simulink model "ALGO_Tanker_new_5Pin_baseline"  (R2023a)
settings: Solver=VariableStepAuto  StartTime=0  StopTime=60  RelTol=1e-3
StopFcn:
  | CompareSimResult_baseline
libraries: simulink x18, Solver_SF x1
(part 1 of 2)
CloseFcn:
  | rollover_simResult_save
settings Model: Creator=QXJ  LastModifiedBy=28303
settings SolverCC: AlgebraicLoopSolver=TrustRegion
settings DebuggingCC: UnconnectedInputMsg=warning  UnconnectedOutputMsg=warning  UnconnectedLineMsg=warning
settings ModelReferenceCC: EnableRefExpFcnMdlSchedulingChecks=on
settings SFSimCC: CustomCodeUndefinedFunction=UseInterfaceOnly

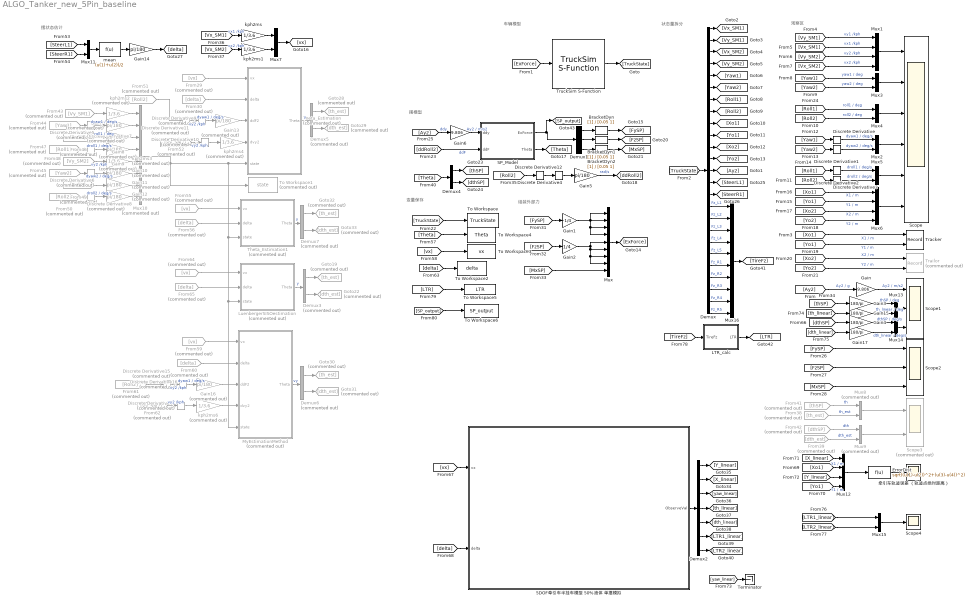
== system ALGO_Tanker_new_5Pin_baseline ==
  note: 摆状态估计
  note: 观察区
  note: 组装外部力
  note: 车辆模型
  note: 状态量拆分
  note: 变量保存
  note: 摆模型
  5DOF牵引车半挂车模型 50%液体 单摆模拟 : Subsystem
  BracketDyn : TransferFcn  Denominator=[0.05 1]
  BracketDyn1 : TransferFcn  Denominator=[0.05 1]
  BracketDyn2 : TransferFcn  Denominator=[0.05 1]
  Demux : Demux  Outputs=25
  Demux1 : Demux  Outputs=3
  Demux2 : Demux  Outputs=7
  Demux{3,5..7} (4 alike) : Demux  Commented=on  Outputs=2
  Demux4 : Demux  Outputs=2
  Discrete Derivative{,1..4,12} (6 alike) : simulink/Discrete/Discrete Derivative  gainval=1.0  ICPrevScaledInput=0.0  OutMin=[]  OutMax=[]  OutDataType=fixdt(1, 16)  OutScaling=2^-10  DoSatur=off
  Discrete Derivative{5..11,15..17} (10 alike) : simulink/Discrete/Discrete Derivative  Commented=on  gainval=1.0  ICPrevScaledInput=0.0  OutMin=[]  OutMax=[]  OutDataType=fixdt(1, 16)  OutScaling=2^-10  DoSatur=off
  ErrorDist : Fcn  Expr=sqrt((u(1)-u(2))^2+(u(3)-u(4))^2)
  From{29,55,59,64} (4 alike) : From  Commented=on  GotoTag=vx
  From{30,56,60,65} (4 alike) : From  Commented=on  GotoTag=delta
  From38 : From  Commented=on  GotoTag=th_est
  From39 : From  Commented=on  GotoTag=dth_est
  From41 : From  Commented=on  GotoTag=thSP
  From42 : From  Commented=on  GotoTag=dthSP
  From43 : From  Commented=on  GotoTag=Vy_SM1
  From44 : From  Commented=on  GotoTag=Yaw1
  From45 : From  Commented=on  GotoTag=Yaw2
  From46 : From  Commented=on  GotoTag=Roll1
  From47 : From  Commented=on  GotoTag=Roll1
  From48 : From  Commented=on  GotoTag=Vy_SM2
  From{49..51,61} (4 alike) : From  Commented=on  GotoTag=Roll2
  From52 : From  Commented=on  GotoTag=Vy_SM2
  From62 : From  Commented=on  GotoTag=Vy_SM2
  Gain : Gain  Gain=9.806
  Gain1 : Gain  Gain=-1/4
  Gain{7..13,16} (8 alike) : Gain  Commented=on  Gain=pi/180
  Gain14 : Gain  Gain=pi/180
  Gain{3..4,15,17} (4 alike) : Gain  Gain=180/pi
  Gain2 : Gain  Gain=1/4
  Gain5 : Gain  Gain=pi/180
  Gain6 : Gain  Gain=9.806
  Goto{19,28,30,32} (4 alike) : Goto  Commented=on  GotoTag=th_est
  Goto{22,29,31,33} (4 alike) : Goto  Commented=on  GotoTag=dth_est
  "LTR_calc " : MATLAB Function  TreatAsAtomicUnit=on
  LuenbergerSISOestimation : MATLAB Function  Commented=on  TreatAsAtomicUnit=on  SystemSampleTime=0.005
  Mux : Mux  Inputs=9
  Mux1 : Mux
  Mux10 : Mux  Commented=on  Inputs=8
  Mux{2..5,7,11,13..15} (9 alike) : Mux  Inputs=2
  Mux12 : Mux
  Mux16 : Mux  Inputs=10
  Mux6 : Mux
  Mux8 : Mux  Commented=on  Inputs=2
  Mux9 : Mux  Commented=on  Inputs=2
  MyEstimationMethod : MATLAB Function  Commented=on  TreatAsAtomicUnit=on  SystemSampleTime=0.005
  SP_Model : MATLAB Function  TreatAsAtomicUnit=on  SystemSampleTime=0.005
  Scope : Scope  NumInputPorts=6
  Scope1 : Scope  NumInputPorts=3
  Scope2 : Scope  NumInputPorts=3
  Scope3 : Scope  Commented=on  NumInputPorts=2
  Scope4 : Scope
  Terminator : Terminator
  Theta_Estimation : MATLAB Function  Commented=on  TreatAsAtomicUnit=on  SystemSampleTime=0.005
  Theta_Estimation1 : MATLAB Function  Commented=on  TreatAsAtomicUnit=on  SystemSampleTime=0.005
  To Workspace : ToWorkspace  VariableName=TruckState  SaveFormat=Timeseries  SampleTime=-1
  To Workspace1 : ToWorkspace  Commented=on  VariableName=state  SaveFormat=Timeseries  SampleTime=-1
  To Workspace2 : ToWorkspace  VariableName=delta  SaveFormat=Timeseries  SampleTime=-1
  To Workspace3 : ToWorkspace  VariableName=vx  SaveFormat=Timeseries  SampleTime=-1
  To Workspace4 : ToWorkspace  VariableName=Theta  SaveFormat=Timeseries  SampleTime=-1
  To Workspace5 : ToWorkspace  VariableName=LTR  SaveFormat=Timeseries  SampleTime=-1
  To Workspace6 : ToWorkspace  VariableName=SP_output  SaveFormat=Timeseries  SampleTime=-1
  Tracker : Record  FileSettingsInternal="{\"entries\":[{\"content\":{\"excelSettings\":{\"content\":{},\"type\":\"Streamout.ExcelSettings\"}},\"type\":\"Streamout.FileSettingStorage\",\"uuid\":\"aec428b3-b5ab-4f46-9125-b809af92a2bd\"}],\"packageUris\":[\"http://schema.mathworks.com/mf0/streamout_blocks/R2020a\"],\"version\":\"1.0\"}"  Layout=[1 1]  SignalsInternal="{\"entries\":[{\"content\":{\"signals\":[{\"content\":{\"blockPath\":[\"ALGO_Tanker_new_5Pin_baseline/Tracker\"],\"dimensions\":[1],\"domain\":\"ALGO_Tanker_new_5Pin_baseline/Tracker\",\"lineColor\":\"#a2142f\",\"plots\":[1],\"port\":1,\"sid\":[\"\"],\"signalID\":43,\"signalName\":\"X1 / m\"},\"type\":\"RecordBlkView.Signal\",\"uuid\":\"2f24ed56-e542-44bd-9784-fd43ced1a2ad\"},{\"content\":{\"blockPath\":[\"ALGO_Tanker_new_5Pin_baseline/Tracker\"],\"dimensions\":[1],\"domain\":\"ALGO_Tanker_new_5Pin_baseline/Tracker\",\"lineColor\":\"#139fff\",\"plots\":[1],\"port\":2,\"sid\":[\"\"],\"signalID\":47,\"signalName\":\"Y1 / m\"},\"type\":\"RecordBlkView.Signal\",\"uuid\":\"888b204b-f2f9-4a07-96ff-cc8a97ec0ab5\"}]},\"type\":\"RecordBlkView.InputSignals\",\"uuid\":\"7c72470c-5bbd-4b03-8b7f-21986a83b27f\"}],\"packageUris\":[\"http://schema.mathworks.com/mf0/streamout_blocks/R2020a\"],\"version\":\"1.0\"}"  VisualizationBindings="{\"xyplotplugin\":{\"info\":[{\"series\":[{\"bindingParametersList\":[{\"parameter\":\"X-Axis\",\"signalID\":43,\"signalName\":\"X1 \\/ m\"},{\"parameter\":\"Y-Axis\",\"signalID\":47,\"signalName\":\"Y1 \\/ m\"}],\"seriesID\":53818}],\"subplotID\":1}]}}"  CompatibilityTag=XY  st=-1
  "Trailor " : Record  Commented=on  FileSettingsInternal="{\"entries\":[{\"content\":{\"excelSettings\":{\"content\":{},\"type\":\"Streamout.ExcelSettings\"}},\"type\":\"Streamout.FileSettingStorage\",\"uuid\":\"42628413-2d8a-4dd7-9eb9-f9d26bce181c\"}],\"packageUris\":[\"http://schema.mathworks.com/mf0/streamout_blocks/R2020a\"],\"version\":\"1.0\"}"  Layout=[1 1]  SignalsInternal="{\"entries\":[{\"content\":{\"signals\":[{\"content\":{\"blockPath\":[\"ALGO_Tanker_new_5Pin_baseline/Trailor \"],\"dimensions\":[1],\"domain\":\"ALGO_Tanker_new_5Pin_baseline/Trailor \",\"lineColor\":\"#a2142f\",\"plots\":[1],\"port\":1,\"signalID\":16,\"signalName\":\"XY Graph:1\"},\"type\":\"RecordBlkView.Signal\",\"uuid\":\"6eea8f1e-a60b-4ba3-9267-a76fcc0df810\"},{\"content\":{\"blockPath\":[\"ALGO_Tanker_new_5Pin_baseline/Trailor \"],\"dimensions\":[1],\"domain\":\"ALGO_Tanker_new_5Pin_baseline/Trailor \",\"lineColor\":\"#139fff\",\"plots\":[1],\"port\":2,\"signalID\":19,\"signalName\":\"XY Graph:2\"},\"type\":\"RecordBlkView.Signal\",\"uuid\":\"9742e65f-64c3-4077-a878-ddc600cf04b1\"}]},\"type\":\"RecordBlkView.InputSignals\",\"uuid\":\"861e839e-7f05-49b0-87d7-e6303be47602\"}],\"packageUris\":[\"http://schema.mathworks.com/mf0/streamout_blocks/R2020a\"],\"version\":\"1.0\"}"  VisualizationBindings="{\"xyplotplugin\":{\"info\":[{\"series\":[{\"bindingParametersList\":[{\"parameter\":\"X-Axis\",\"signalID\":16,\"signalName\":\"XY Graph:1\"},{\"parameter\":\"Y-Axis\",\"signalID\":19,\"signalName\":\"XY Graph:2\"}],\"seriesID\":50861}],\"subplotID\":1}]}}"  CompatibilityTag=XY  st=-1
  TruckSim S-Function : Solver_SF/TruckSim S-Function  Priority=1  SIMFILE=ALGO_Tanker_TrajTrack_5Pin_Baseline.sim
      settings: SourceProductName=TruckSim S-Function
  kph2ms : Gain  Gain=1/3.6
  kph2ms1 : Gain  Gain=1/3.6
  kph2ms{2..4,6} (4 alike) : Gain  Commented=on  Gain=1/3.6
  mean : Fcn  Expr=(u(1)+u(2))/2
  牵引车轨迹误差 （轨迹点绝对距离） : Scope
  wires:
  kph2ms1/1 -> Mux7/2
  Mux7/1 -> [vx]
  kph2ms/1 -> Mux7/1
  From30/1 -> Theta_Estimation/2(delta)
  From29/1 -> Theta_Estimation/1(vx)
  [Vx_SM1] -> kph2ms/1  "vx1 /kph"
  [Vx_SM2] -> kph2ms1/1  "vx2 /kph"
  From45/1 -> Discrete Derivative6/1
  Discrete Derivative7/1 -> Gain9/1  "droll1 / deg/s"
  From47/1 -> Discrete Derivative7/1
  From50/1 -> Discrete Derivative8/1
  From43/1 -> kph2ms2/1
  From48/1 -> kph2ms3/1  "vy2 /kph"
  From44/1 -> Discrete Derivative5/1
  Discrete Derivative5/1 -> Gain7/1  "dyaw1 / deg/s"
  From46/1 -> Gain8/1  "roll1 / deg"
  Discrete Derivative6/1 -> Gain10/1  "dyaw2 / deg/s"
  From49/1 -> Gain11/1
  Discrete Derivative8/1 -> Gain12/1  "droll2 / deg/s"
  Gain12/1 -> Mux10/8
  Gain11/1 -> Mux10/7
  Gain10/1 -> Mux10/6
  kph2ms3/1 -> Mux10/5
  Gain9/1 -> Mux10/4
  Gain8/1 -> Mux10/3
  Gain7/1 -> Mux10/2
  kph2ms2/1 -> Mux10/1
  Discrete Derivative9/1 -> Gain13/1  "dyaw1 / deg/s"
  Discrete Derivative11/1 -> Discrete Derivative9/1  "vy2 /kph"
  From52/1 -> Discrete Derivative10/1  "vy2 /kph"
  Discrete Derivative10/1 -> kph2ms4/1
  From51/1 -> Discrete Derivative11/1
  Gain13/1 -> Theta_Estimation/3(ddF2)
  kph2ms4/1 -> Theta_Estimation/4(dvy2)
  [SteerL1] -> Mux11/1
  Mux11/1 -> mean/1
  [SteerR1] -> Mux11/2
  mean/1 -> Gain14/1
  Gain14/1 -> [delta]
  From55/1 -> Theta_Estimation1/1(vx)
  From56/1 -> Theta_Estimation1/2(delta)
  kph2ms6/1 -> MyEstimationMethod/4(dvy2)
  From62/1 -> Discrete Derivative17/1  "vy2 /kph"
  Discrete Derivative17/1 -> kph2ms6/1
  From61/1 -> Discrete Derivative15/1
  Gain16/1 -> MyEstimationMethod/3(ddF2)
  Discrete Derivative16/1 -> Gain16/1  "dyaw1 / deg/s"
  Discrete Derivative15/1 -> Discrete Derivative16/1  "vy2 /kph"
  From60/1 -> MyEstimationMethod/2(delta)
  From59/1 -> MyEstimationMethod/1(vx)
  Mux10/1 -> To Workspace1/1, Theta_Estimation/5(state), LuenbergerSISOestimation/3(state), MyEstimationMethod/5(state), Theta_Estimation1/3(state)
  MyEstimationMethod/1(Theta) -> Demux6/1  "vy"
  Demux3/1 -> Goto19/1
  Demux3/2 -> Goto22/1
  From64/1 -> LuenbergerSISOestimation/1(vx)
  From65/1 -> LuenbergerSISOestimation/2(delta)
  Theta_Estimation1/1(Theta) -> Demux7/1  "y"
  Demux5/2 -> Goto29/1
  Demux5/1 -> Goto28/1
  Theta_Estimation/1(Theta) -> Demux5/1  "y"
  LuenbergerSISOestimation/1(Theta) -> Demux3/1  "y"
  Demux6/2 -> Goto31/1
  Demux6/1 -> Goto30/1
  Demux7/2 -> Goto33/1
  Demux7/1 -> Goto32/1
  Discrete Derivative/1 -> Mux2/1  "dyaw1 / deg/s"
  Demux/12 -> [Yo2]
  Demux/11 -> [Xo2]
  [Xo1] -> Mux6/1  "X1 / m"
  TruckSim S-Function/1 -> [TruckState]
  [Xo2] -> "Trailor "/1  "X2 / m"
  Demux/1 -> [Vx_SM1]
  [TruckState] -> Demux/1
  [Yaw1] -> Mux3/1  "yaw1 / deg"
  [Yaw2] -> Mux3/2  "yaw2 / deg"
  Mux5/1 -> Scope/5
  Gain1/1 -> Mux/1, Mux/4, Mux/3, Mux/2
  [MxSP] -> Scope2/3
  [thSP] -> Gain3/1
  SP_Model/2(Theta) -> [Theta]
  Gain6/1 -> SP_Model/1(ddy)  "Ay2 / m/s2"
  [Vy_SM2] -> Mux1/3  "vy2 /kph"
  [Roll2] -> Mux4/2  "roll2 / deg"
  From39/1 -> Mux9/2  "dth_est"
  Demux4/1 -> [thSP]
  From38/1 -> Mux8/2  "th_est"
  Demux1/2 -> BracketDyn1/1
  Mux1/1 -> Scope/1
  [Theta] -> Demux4/1
  Demux/3 -> [Vx_SM2]
  Demux4/2 -> [dthSP]
  [Roll1] -> Mux4/1  "roll1 / deg"
  Mux4/1 -> Scope/3
  Gain4/1 -> Mux14/1  "dthSP / deg/s"
  BracketDyn/1 -> [FySP]
  BracketDyn1/1 -> [FzSP]
  Demux/2 -> [Vy_SM1]
  Gain5/1 -> [ddRoll2]  "rad/s"
  [Ay2] -> Gain6/1  "ddy"
  Discrete Derivative4/1 -> Discrete Derivative12/1
  [Roll2] -> Discrete Derivative4/1
  [Vx_SM2] -> Mux1/4  "vx2 /kph"
  [FySP] -> Gain1/1
  [Yaw1] -> Discrete Derivative/1
  SP_Model/1(ExForce) -> [SP_output], Demux1/1
  [Yo1] -> Mux6/2  "Y1 / m"
  [Roll1] -> Discrete Derivative2/1
  [Vx_SM1] -> Mux1/2  "vx1 /kph"
  Demux/9 -> [Xo1]
  [FzSP] -> Scope2/2
  [Yaw2] -> Discrete Derivative1/1
  [ExForce] -> TruckSim S-Function/1
  Demux1/1 -> BracketDyn/1
  Discrete Derivative2/1 -> Mux5/1  "droll1 / deg/s"
  From41/1 -> Mux8/1  "th"
  BracketDyn2/1 -> [MxSP]
  Demux/14 -> [SteerL1]
  Mux/1 -> [ExForce]
  [Roll2] -> Discrete Derivative3/1
  Mux6/1 -> Scope/6
  [Xo1] -> Tracker/1  "X1 / m"
  Demux/21 -> Mux16/6  "Fz_R1"
  Demux/22 -> Mux16/7  "Fz_R2"
  "LTR_calc "/1(LTR) -> [LTR]
  Mux9/1 -> Scope3/2
  Gain17/1 -> Mux14/2  "dth_linear / deg/s"
  Gain/1 -> Scope1/1  "Ay2 / m/s2"
  [TireFz] -> "LTR_calc "/1(TireFz)
  Demux/13 -> [Ay2]
  Demux/19 -> Mux16/4  "Fz_L4"
  Demux2/4 -> [th_linear]
  [dth_linear] -> Gain17/1
  Mux15/1 -> Scope4/1
  [Yo1] -> Tracker/2  "Y1 / m"
  Demux2/1 -> [Y_linear]
  Demux2/6 -> [LTR1_linear]
  5DOF牵引车半挂车模型 50%液体 单摆模拟/1(ObserveVal) -> Demux2/1
  [ddRoll2] -> SP_Model/2(ddF)  "ddF"
  Mux14/1 -> Scope1/3
  [yaw_linear] -> Terminator/1
  Mux2/1 -> Scope/4
  [Xo1] -> Mux12/2  "X1 / m"
  [Theta] -> To Workspace4/1
  [th_linear] -> Gain15/1
  Mux12/1 -> ErrorDist/1
  Demux/10 -> [Yo1]
  [Y_linear] -> Mux12/3
  Mux8/1 -> Scope3/1
  Demux2/7 -> [LTR2_linear]
  Demux/15 -> [SteerR1]
  Mux3/1 -> Scope/2
  Demux/6 -> [Yaw2]
  [Xo2] -> Mux6/3  "X2 / m"
  Demux2/2 -> [X_linear]
  [vx] -> To Workspace3/1
  [MxSP] -> Mux/9
  Demux/4 -> [Vy_SM2]
  Demux2/5 -> [dth_linear]
  [delta] -> 5DOF牵引车半挂车模型 50%液体 单摆模拟/2("delta ")
  Demux/7 -> [Roll1]
  [LTR2_linear] -> Mux15/2
  [dthSP] -> Gain4/1
  [vx] -> 5DOF牵引车半挂车模型 50%液体 单摆模拟/1(vx)
  [delta] -> To Workspace2/1
  Mux13/1 -> Scope1/2
  [Vy_SM1] -> Mux1/1  "vy1 /kph"
  [X_linear] -> Mux12/1
  ErrorDist/1 -> 牵引车轨迹误差 （轨迹点绝对距离）/1
  From42/1 -> Mux9/1  "dth"
  [Yo2] -> "Trailor "/2  "Y2 / m"
  [SP_output] -> To Workspace6/1
  Gain3/1 -> Mux13/1  "thSP / deg"
  Demux/8 -> [Roll2]
  Mux16/1 -> [TireFz]
  Gain15/1 -> Mux13/2  "th_linear / deg"
  [FzSP] -> Gain2/1
  Demux/5 -> [Yaw1]
  [Ay2] -> Gain/1  "Ay2 / g"
  Demux/17 -> Mux16/2  "Fz_L2"
  [Yo2] -> Mux6/4  "Y2 / m"
  Discrete Derivative1/1 -> Mux2/2  "dyaw2 / deg/s"
  [Yo1] -> Mux12/4  "Y1 / m"
  [LTR] -> To Workspace5/1
  [LTR1_linear] -> Mux15/1
  [FySP] -> Scope2/1
  Discrete Derivative3/1 -> Mux5/2  "droll2 / deg/s"
  Demux/16 -> Mux16/1  "Fz_L1"
  Demux1/3 -> BracketDyn2/1
  Discrete Derivative12/1 -> Gain5/1
  Gain2/1 -> Mux/8, Mux/7, Mux/6, Mux/5
  Demux/24 -> Mux16/9  "Fz_R4"
  Demux/20 -> Mux16/5  "Fz_L5"
  Demux/23 -> Mux16/8  "Fz_R3"
  Demux/18 -> Mux16/3  "Fz_L3"
  Demux2/3 -> [yaw_linear]
  Demux/25 -> Mux16/10  "Fz_R5"
  [TruckState] -> To Workspace/1

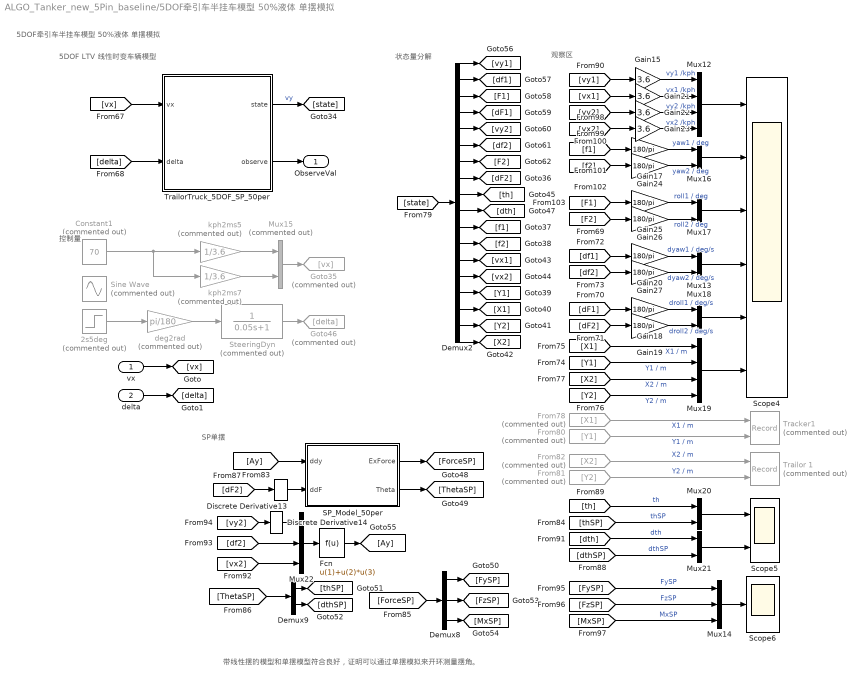
== system ALGO_Tanker_new_5Pin_baseline/5DOF牵引车半挂车模型 50%液体 单摆模拟 ==
  note: SP单摆
  note: 带线性摆的模型和单摆模型符合良好，证明可以通过单摆模拟来开环测量摆角。
  note: 控制量
  note: 5DOF牵引车半挂车模型 50%液体 单摆模拟
  note: 状态量分解
  note: 5DOF LTV 线性时变车辆模型
  note: 观察区
  vx : Inport
  "delta " : Inport  Port=2
  2s5deg : Step  Commented=on  Time=2  After=5  SampleTime=0
  Constant1 : Constant  Commented=on  Value=70
  Demux2 : Demux  Outputs=18
  Demux8 : Demux  Outputs=3
  Demux9 : Demux  Outputs=2
  Discrete Derivative13 : simulink/Discrete/Discrete Derivative  gainval=1.0  ICPrevScaledInput=0.0  OutMin=[]  OutMax=[]  OutDataType=fixdt(1, 16)  OutScaling=2^-10  DoSatur=off
  Discrete Derivative14 : simulink/Discrete/Discrete Derivative  gainval=1.0  ICPrevScaledInput=0.0  OutMin=[]  OutMax=[]  OutDataType=fixdt(1, 16)  OutScaling=2^-10  DoSatur=off
  Fcn : Fcn  Expr=u(1)+u(2)*u(3)
  From78 : From  Commented=on  GotoTag=X1
  From80 : From  Commented=on  GotoTag=Y1
  From81 : From  Commented=on  GotoTag=Y2
  From82 : From  Commented=on  GotoTag=X2
  Gain{15,21..23} (4 alike) : Gain  Gain=3.6
  Gain{17..20,24..27} (8 alike) : Gain  Gain=180/pi
  Goto35 : Goto  Commented=on  GotoTag=vx
  Goto46 : Goto  Commented=on  GotoTag=delta
  Mux12 : Mux
  Mux{13,16..18,20..21} (6 alike) : Mux  Inputs=2
  Mux14 : Mux  Inputs=3
  Mux15 : Mux  Commented=on  Inputs=2
  Mux19 : Mux
  Mux22 : Mux  Inputs=3
  SP_Model_50per : MATLAB Function  TreatAsAtomicUnit=on  SystemSampleTime=0.005
  Scope4 : Scope  NumInputPorts=6
  Scope5 : Scope  NumInputPorts=2
  Scope6 : Scope
  Sine Wave : Sin  Commented=on  Amplitude=25  Frequency=2*pi*0.2  SampleTime=0
  SteeringDyn : TransferFcn  Commented=on  Denominator=[0.05 1]
  Tracker1 : Record  Commented=on  FileSettingsInternal="{\"entries\":[{\"content\":{\"excelSettings\":{\"content\":{},\"type\":\"Streamout.ExcelSettings\"}},\"type\":\"Streamout.FileSettingStorage\",\"uuid\":\"a90f987a-d528-48a3-b948-a80540f660a2\"}],\"packageUris\":[\"http://schema.mathworks.com/mf0/streamout_blocks/R2020a\"],\"version\":\"1.0\"}"  Layout=[1 1]  SignalsInternal="{\"entries\":[{\"content\":{\"signals\":[{\"content\":{\"blockPath\":[\"ALGO_Tanker_new_5Pin_baseline/5DOF牵引车半挂车模型 50%液体 单摆模拟/Tracker1\"],\"dimensions\":[1],\"domain\":\"ALGO_Tanker_new_5Pin_baseline/5DOF￧ﾉﾵ￥ﾼﾕ￨ﾽﾦ￥ﾍﾊ￦ﾌﾂ￨ﾽﾦ￦ﾨﾡ￥ﾞﾋ 50%￦ﾶﾲ￤ﾽﾓ ￥ﾍﾕ￦ﾑﾆ￦ﾨﾡ￦ﾋﾟ/Tracker1\",\"lineColor\":\"#a2142f\",\"plots\":[1],\"port\":1,\"signalID\":24,\"signalName\":\"XY Graph:1\"},\"type\":\"RecordBlkView.Signal\",\"uuid\":\"3ed66f4e-d292-443a-9652-1644885d5cf5\"},{\"content\":{\"blockPath\":[\"ALGO_Tanker_new_5Pin_baseline/5DOF牵引车半挂车模型 50%液体 单摆模拟/Tracker1\"],\"dimensions\":[1],\"domain\":\"ALGO_Tanker_new_5Pin_baseline/5DOF￧ﾉﾵ￥ﾼﾕ￨ﾽﾦ￥ﾍﾊ￦ﾌﾂ￨ﾽﾦ￦ﾨﾡ￥ﾞﾋ 50%￦ﾶﾲ￤ﾽﾓ ￥ﾍﾕ￦ﾑﾆ￦ﾨﾡ￦ﾋﾟ/Tracker1\",\"lineColor\":\"#139fff\",\"plots\":[1],\"port\":2,\"signalID\":27,\"signalName\":\"XY Graph:2\"},\"type\":\"RecordBlkView.Signal\",\"uuid\":\"03e0ba51-6389-48fb-8d2a-e503b4cbd9e5\"}]},\"type\":\"RecordBlkView.InputSignals\",\"uuid\":\"2c6dba3d-ae40-4061-a45b-5c20937c901b\"}],\"packageUris\":[\"http://schema.mathworks.com/mf0/streamout_blocks/R2020a\"],\"version\":\"1.0\"}"  VisualizationBindings="{\"xyplotplugin\":{\"info\":[{\"series\":[{\"bindingParametersList\":[{\"parameter\":\"X-Axis\",\"signalID\":24,\"signalName\":\"XY Graph:1\"},{\"parameter\":\"Y-Axis\",\"signalID\":27,\"signalName\":\"XY Graph:2\"}],\"seriesID\":47850}],\"subplotID\":1}]}}"  CompatibilityTag=XY  st=-1
  Trailor 1 : Record  Commented=on  FileSettingsInternal="{\"entries\":[{\"content\":{\"excelSettings\":{\"content\":{},\"type\":\"Streamout.ExcelSettings\"}},\"type\":\"Streamout.FileSettingStorage\",\"uuid\":\"ee976611-5a1b-436c-9467-2f509ccfb164\"}],\"packageUris\":[\"http://schema.mathworks.com/mf0/streamout_blocks/R2020a\"],\"version\":\"1.0\"}"  Layout=[1 1]  SignalsInternal="{\"entries\":[{\"content\":{\"signals\":[{\"content\":{\"blockPath\":[\"ALGO_Tanker_new_5Pin_baseline/5DOF牵引车半挂车模型 50%液体 单摆模拟/Trailor 1\"],\"dimensions\":[1],\"domain\":\"ALGO_Tanker_new_5Pin_baseline/5DOF￧ﾉﾵ￥ﾼﾕ￨ﾽﾦ￥ﾍﾊ￦ﾌﾂ￨ﾽﾦ￦ﾨﾡ￥ﾞﾋ 50%￦ﾶﾲ￤ﾽﾓ ￥ﾍﾕ￦ﾑﾆ￦ﾨﾡ￦ﾋﾟ/Trailor 1\",\"lineColor\":\"#a2142f\",\"plots\":[1],\"port\":1,\"signalID\":32,\"signalName\":\"XY Graph:1\"},\"type\":\"RecordBlkView.Signal\",\"uuid\":\"54d57959-15ed-4e42-bd0f-8cbd995d0bf1\"},{\"content\":{\"blockPath\":[\"ALGO_Tanker_new_5Pin_baseline/5DOF牵引车半挂车模型 50%液体 单摆模拟/Trailor 1\"],\"dimensions\":[1],\"domain\":\"ALGO_Tanker_new_5Pin_baseline/5DOF￧ﾉﾵ￥ﾼﾕ￨ﾽﾦ￥ﾍﾊ￦ﾌﾂ￨ﾽﾦ￦ﾨﾡ￥ﾞﾋ 50%￦ﾶﾲ￤ﾽﾓ ￥ﾍﾕ￦ﾑﾆ￦ﾨﾡ￦ﾋﾟ/Trailor 1\",\"lineColor\":\"#139fff\",\"plots\":[1],\"port\":2,\"signalID\":35,\"signalName\":\"XY Graph:2\"},\"type\":\"RecordBlkView.Signal\",\"uuid\":\"095e148a-9d51-41f4-bd97-85008a41f26b\"}]},\"type\":\"RecordBlkView.InputSignals\",\"uuid\":\"4401373d-b9f0-4087-a766-ee8aa40abb39\"}],\"packageUris\":[\"http://schema.mathworks.com/mf0/streamout_blocks/R2020a\"],\"version\":\"1.0\"}"  VisualizationBindings="{\"xyplotplugin\":{\"info\":[{\"series\":[{\"bindingParametersList\":[{\"parameter\":\"X-Axis\",\"signalID\":32,\"signalName\":\"XY Graph:1\"},{\"parameter\":\"Y-Axis\",\"signalID\":35,\"signalName\":\"XY Graph:2\"}],\"seriesID\":49081}],\"subplotID\":1}]}}"  CompatibilityTag=XY  st=-1
  TrailorTruck_5DOF_SP_50per : MATLAB Function  TreatAsAtomicUnit=on  SystemSampleTime=0.01
  deg2rad : Gain  Commented=on  Gain=pi/180
  kph2ms5 : Gain  Commented=on  Gain=1/3.6
  kph2ms7 : Gain  Commented=on  Gain=1/3.6
  ObserveVal : Outport  VectorParamsAs1DForOutWhenUnconnected=off
  wires:
  Demux2/17 -> [Y2]
  [vx2] -> Mux22/3
  [vx1] -> Gain21/1
  [FzSP] -> Mux14/2  "FzSP"
  Mux16/1 -> Scope4/2
  Gain25/1 -> Mux17/1  "roll1 / deg"
  Mux17/1 -> Scope4/3
  [Y1] -> Mux19/2  "Y1 / m"
  [vy2] -> Gain22/1
  [state] -> Demux2/1
  From78/1 -> Tracker1/1  "X1 / m"
  Demux2/9 -> [th]
  [MxSP] -> Mux14/3  "MxSP"
  Demux2/18 -> [X2]
  Gain26/1 -> Mux17/2  "roll2 / deg"
  From81/1 -> Trailor 1/2  "Y2 / m"
  Mux14/1 -> Scope6/1
  Gain21/1 -> Mux12/2  "vx1 /kph"
  SteeringDyn/1 -> Goto46/1
  [dF2] -> Gain19/1
  [f2] -> Gain24/1
  [dF1] -> Gain18/1
  [vx2] -> Gain23/1
  [F2] -> Gain26/1
  Demux2/7 -> [F2]
  From80/1 -> Tracker1/2  "Y1 / m"
  Demux2/14 -> [vx2]
  Demux2/11 -> [f1]
  Gain27/1 -> Mux13/2  "dyaw2 / deg/s"
  [df1] -> Gain20/1
  2s5deg/1 -> deg2rad/1
  [F1] -> Gain25/1
  [X1] -> Mux19/1  "X1 / m"
  Gain19/1 -> Mux18/2  "droll2 / deg/s"
  Gain18/1 -> Mux18/1  "droll1 / deg/s"
  Mux19/1 -> Scope4/6
  Demux8/3 -> [MxSP]
  [df2] -> Mux22/2
  Discrete Derivative14/1 -> Mux22/1
  Mux20/1 -> Scope5/1
  Gain15/1 -> Mux12/1  "vy1 /kph"
  Mux13/1 -> Scope4/4
  Gain23/1 -> Mux12/4  "vx2 /kph"
  [FySP] -> Mux14/1  "FySP"
  [vy1] -> Gain15/1
  Demux2/4 -> [dF1]
  Fcn/1 -> [Ay]
  Mux22/1 -> Fcn/1
  kph2ms5/1 -> Mux15/1
  [ThetaSP] -> Demux9/1
  Mux15/1 -> Goto35/1
  [dthSP] -> Mux21/2  "dthSP"
  [thSP] -> Mux20/2  "thSP"
  deg2rad/1 -> SteeringDyn/1
  Gain24/1 -> Mux16/2  "yaw2 / deg"
  Demux2/12 -> [f2]
  [X2] -> Mux19/3  "X2 / m"
  Discrete Derivative13/1 -> SP_Model_50per/2(ddF)
  Demux8/1 -> [FySP]
  Demux8/2 -> [FzSP]
  Gain17/1 -> Mux16/1  "yaw1 / deg"
  Gain20/1 -> Mux13/1  "dyaw1 / deg/s"
  [vy2] -> Discrete Derivative14/1
  Mux18/1 -> Scope4/5
  [ForceSP] -> Demux8/1
  SP_Model_50per/1(ExForce) -> [ForceSP]
  TrailorTruck_5DOF_SP_50per/1(state) -> [state]  "vy"
  [delta] -> TrailorTruck_5DOF_SP_50per/2(delta)
  [dF2] -> Discrete Derivative13/1
  [f1] -> Gain17/1
  Demux2/15 -> [Y1]
  Mux12/1 -> Scope4/1
  [vx] -> TrailorTruck_5DOF_SP_50per/1(vx)
  From82/1 -> Trailor 1/1  "X2 / m"
  Demux2/6 -> [df2]
  Demux2/2 -> [df1]
  kph2ms7/1 -> Mux15/2
  Demux2/5 -> [vy2]
  Demux2/3 -> [F1]
  [Ay] -> SP_Model_50per/1(ddy)
  SP_Model_50per/2(Theta) -> [ThetaSP]
  Demux2/8 -> [dF2]
  Demux9/1 -> [thSP]
  [Y2] -> Mux19/4  "Y2 / m"
  Demux2/16 -> [X1]
  Constant1/1 -> kph2ms7/1, kph2ms5/1
  Demux2/13 -> [vx1]
  Demux2/1 -> [vy1]
  Demux9/2 -> [dthSP]
  [df2] -> Gain27/1
  Mux21/1 -> Scope5/2
  [dth] -> Mux21/1  "dth"
  [th] -> Mux20/1  "th"
  Demux2/10 -> [dth]
  Gain22/1 -> Mux12/3  "vy2 /kph"
  vx/1 -> [vx]
  "delta "/1 -> [delta]
  TrailorTruck_5DOF_SP_50per/2(observe) -> ObserveVal/1

== matlab function ALGO_Tanker_new_5Pin_baseline/SP_Model ==
  data: ddy input; ExForce output; ddF input; Theta output
function [ExForce,Theta] = SP_Model(ddy,ddF)
persistent sim_param Ts y0
%% 定义摆
if isempty(Ts)
%SP模型，共5个参数拟合
% 参数 m1 h0 hp lp coeff
x=[10890,1.5,0.13,0.97,0.13];
% 获取参数
sim_param=getParam_SP(x);
%初始状态量
y0=zeros(9,1);
%采样时间
Ts=0.005;
end

y=y0;

%% 求解微分方程
dy=zeros(9,1);
dy(1)=y(2);
dy(2)=ddy;
dy(3)=(dy(2)-y(3))/Ts;
dy(4)=y(5);
dy(5)=ddF;
dy(6)=(dy(5)-y(6))/Ts;
dy(7)=y(8);
dy(8)=calc_ddth_SP(y,sim_param);
dy(9)=(dy(8)-y(9))/Ts;
y=y0+dy*Ts;
%% 计算三向力输出
[Fy,Fz,Mx]=calc_Fp_SP(y,sim_param);
ExForce=[Fy,Fz,Mx];
%% 更新状态量
y0=y;
th=y(7);
dth=y(8);
Theta=[th,dth];
end

%% 根据变量获取参数
function sim_param=getParam_SP(x)
%根据变量生成传输参数
TotMass=14462;
m1=x(1);%参数1
m0=TotMass-m1;
h0=x(2);%参数2
hp=x(3);%参数3
lp=x(4);%参数4
g=9.806;
coeff=x(5);%参数5
sim_param=[m0,m1,h0,hp,lp,g,coeff];
end

%% 求解三向力输出
function [Fy,Fz,Mx] = calc_Fp_SP(state,param)
% sim_param=[m0,m1,h0,hp,lp,g,coeff];
m0=param(1);
m1=param(2);
h0=param(3);
hp=param(4);
lp=param(5);
g=param(6);
% co=param(7);

% y=state(1);
% dy=state(2);
ddy=state(3);
f=state(4);
df=state(5);
ddf=state(6);
th=state(7);
dth=state(8);
ddth=state(9);

%定义运算符简写
sf=sin(f);
cf=cos(f);
s2=sin(th+f);
c2=cos(th+f);
L=lp+hp;
%定义质量块的 位置矢量
exh=0.77; %额外增加的高度是罐底到车轴心的高度
R0=[-(exh+h0)*sf,(exh+h0)*cf];

R1=[-(exh+L)*sf+lp*s2
    (exh+L)*cf-lp*c2];

ddRp0=[ddy-h0*cf*ddf+df^2*h0*sf
-h0*sf*ddf-h0*cf*df^2+g];

ddRp1=[ddy+ddf*(-L*cf+lp*c2)+ddth*(lp*c2)+df^2*(L*sf-lp*s2)+dth^2*(-lp*s2)+df*dth*(-2*lp*s2)
ddf*(-L*sf+lp*s2)+ddth*(lp*s2)+df^2*(-L*cf+lp*c2)+dth^2*(lp*c2)+df*dth*(2*lp*c2)+g];

Fp=m0*ddRp0+m1*ddRp1;
Fy=Fp(1)*cf-(-Fp(2))*sf;
Fz=(-Fp(2))*cf+Fp(1)*sf;
Mx0=(m0*(R0(1)*-ddRp0(2)+R0(2)*ddRp0(1)));
Mx1=(m1*(R1(1)*-ddRp1(2)+R1(2)*ddRp1(1)));

Mx=Mx0+Mx1;

end
%% 求解ddth
function ddth = calc_ddth_SP(state,param)
% sim_param=[m0,m1,h0,hp,lp,g,coeff];
% m0=param(1);
% m1=param(2);
% h0=param(3);
hp=param(4);
lp=param(5);
g=param(6);
co=param(7);

% y=state(1);
% dy=state(2);
ddy=state(3);
f=state(4);
df=state(5);
ddf=state(6);
th=state(7);
dth=state(8);
% ddth=state(9);


%定义运算符简写
s1=sin(th);
c1=cos(th);
s2=sin(th+f);
c2=cos(th+f);
L=lp+hp;

ddth=-(ddy*lp*c2+ddf*(-lp*L*c1+lp^2)-df^2*lp*L*s1+g*lp*s2)/(lp^2);
ddth=ddth-co*dth;

end

== matlab function ALGO_Tanker_new_5Pin_baseline/Theta_Estimation ==
  data: vx input; delta input; ddF2 input; dvy2 input; state input; Theta output
function Theta=Theta_Estimation(vx,delta,ddF2,dvy2,state)
%% 初始状态定义
%要记得设置本模块的采样时间哦
persistent Ts                             %采样时间
persistent th0 dth0 state0 lambda   %摆状态
if isempty(th0)
    Ts=0.005;
   th0=0;dth0=0; 
   state0=zeros(8,1);
   lambda=0.995;
end
%% 定义动力学模型参数
persistent a b c d e                    %轴距纵向几何参数
persistent h1 h2 hc1 hc2                %质心至侧倾轴线距离
                                        %铰接点至侧倾轴线距离
persistent m1 m2 m1s m2s g;g=9.806;
persistent I1zz I1xx I1xz I2zz I2xx I2xz %惯性参量
persistent k1 k2 k3                      %线性轮胎模型参数
persistent kr1 kr2 c1 c2 k12             %悬架模型参数
persistent m0 mp h0 hp lp co             %摆模型参数
if isempty(a)
%SP模型，共5个参数拟合
% 参数 m1 h0 hp lp coeff
x=[10890,1.5,0.13,0.97,0.13];
sim_param=getParam_SP(x);
% sim_param=[m0,m1,h0+0.77,hp+0.77,lp,g,coeff];
m0=sim_param(1);
mp=sim_param(2);
h0=sim_param(3);
hp=sim_param(4);
lp=sim_param(5);
co=sim_param(7);
%车辆模型参数
L1=(5+6.27)/2;L2=(10.15+11.5)/2;       %轴距平均
a=1.385;b=L1-a;c=5.635-a;e=5.5;d=L2-e; %纵向几何
hm1s=1.02; %牵引车质心高度
hm2s=1.58; %50%充液率时半挂车质心高度
hhitch=1.1;%交接点高度
hroll1=0.2314;hroll2=0.9630;                     %侧倾中心高度
h1=hm1s-hroll1;h2=hm2s-hroll2;hc1=hhitch-hroll1;hc2=hhitch-hroll2;%高度几何
m1s=6310;m1=m1s+570+785*2;             %牵引车质量
% m2s=5925;m2=m2s+665*2;                 %半挂车空载质量
m2s=20387;m2=m2s+665*2;
I1xx=6879;I1xz=130;I1zz=19665;         %牵引车惯量
% I2xx=9960;I2xz=0;I2zz=179992;          %半挂车惯量
I2xx=34652;I2xz=0;I2zz=331380;
%轮胎模型参数
k1=-37e4;k2=-82e4;k3=-80e4;             %侧偏刚度
kr1=18.7e5;kr2=9.14e5;k12=68.3e5;             %侧倾刚度
c1=64.4e3;c2=197.7e3;                        %悬架等效阻尼
end
%% 定义线性动力学模型
df2=state0(6);
dF2=state0(8);
vx1=vx(1);vx2=vx(2);
%线性车辆动力学模型
% M*dX = A0*X + B0*u
m14=-m1s*h1*c-I1xz;
m21=m1*vx1*hc1-m1s*h1*vx1;
m24=I1xx+2*m1s*h1^2-m1s*h1*hc1;
m55=m2*vx2*hc2-m2s*h2*vx2;
m58=I2xx+2*m2s*h2^2-m2s*h2*hc2;

M=[m1*vx1*c, I1zz, 0,   m14,     0,        0,   0,     0;
    m21,    -I1xz, 0,   m24,     0,        0,   0,     0;
   m1*vx1,      0, 0, -m1s*h1, m2*vx2,     0,   0, -m2s*h2;
     0,         0, 0,     0,  m2*vx2*e, -I2zz,  0, I2xz-m2s*h2*e;
     0,         0, 0,     0,    m55,    -I2xz,  0,    m58;
     1,    -c/vx1, 0, -hc1/vx1,  -1,   -e/vx2,  0, hc2/vx2;
     0,         0, 1,     0,     0,        0,   0,     0;
     0,         0, 0,     0,     0,        0,   1,     0   ];
 
 a11 = (c+a)*k1 + (c-b)*k2;
 a12 = a*(c+a)*k1/vx1 - b*(c-b)*k2/vx1 - m1*vx1*c;
 a22 = (a*k1-b*k2)*hc1/vx1 + (m1s*h1-m1*hc1)*vx1;
 a23 = m1s*g*h1 - kr1 -k12;
 a32 = (a*k1-b*k2)/vx1 - m1*vx1;
 a36 = -d*k3/vx2 - m2*vx2;
 a46 = -d*(e+d)*k3/vx2 - m2*vx2*e;
 a56 = (m2s*h2-m2*hc2)*vx2 - d*k3*hc2/vx2;
 a57 = m2s*g*h2 - kr2 -k12;
 %  X=   b1     df1    F1  dF1        b2  df2, F2   dF2 
 Acm0=[ a11,    a12,    0,   0,       0,   0,  0,    0;
   (k1+k2)*hc1, a22,  a23, -c1,       0,   0, k12,   0;
     k1+k2,     a32,    0,   0,      k3,  a36, 0,    0;
        0,       0,     0,   0, (e+d)*k3, a46, 0,    0;
        0,       0,    k12,  0, e*k3*h2, a56, a57, -c2;
        0,      -1,     0,   0,       0,   1,  0,    0;
        0,       0,     0,   1,       0,   0,  0,    0;
        0,       0,     0,   0,       0,   0,  0,    1   ];
    
 Bcm0=[-(c+a)*k1, -k1*hc1, -k1, 0, 0, 0, 0, 0]';

 %       1    2   3    4    5    6    7    8   9   10  11   12   13  14  15 16  17 18
%  X = vy1,  df1,F1, dF1, vy2, df2,  F2, dF2, f1, f2, vx1, vx2, Y1, X1, Y2,X2  th dth
% dX = dvy1;ddf1;dF1;ddF1;dvy2;ddf2;dF2;ddF2;df1;df2;dvx1;dvx2;dY1;dX1;dY2;dX2;dth;ddth
th=th0;dth=dth0;

M_=zeros(10);
M_(10,5)=cos(th)/lp;
M_(10,9)=co;
M_(10,10)=1;
M_(9,9)=1;
M_(3,:)=[0,0,0,0,m0-mp*(cos(th)^2-1),0,0,-h0*m0-mp*(hp+lp-lp),...
    -mp*(co*lp+2*dth*lp*sin(th)),0];
M_(4,:)=M_(3,:)*e;
M_(5,:)=M_(3,:)*hc2+...
[0,0,0,0,-h0*m0-hp*mp*sin(th)^2-lp*mp*sin(th)^2,0,-2*dF2*lp*mp*sin(th)*(hp+lp-lp),...
  m0*h0^2+mp*((hp+lp-lp)^2+lp^2*sin(th)^2),0,0];

%       1    2   3    4    5    6    7    8   17 18
%  X =  0,   0,  0,   0, vy2,   0,  F2, dF2,  th  0
% dX =  0,   0,  0,   0,  0;  ddf2; 0; ddF2;;dth;ddth 
A_=zeros(10);
A_(9,10)=1;
A_(10,6)=-(vx2)/lp;
a_317=mp*(ddF2*lp*sin(th)+(cos(th)*(g*lp-lp*sin(th)*(dvy2+df2*vx2)))...
    /lp+dth^2*lp-lp*sin(th)*(co*dth+(g*lp*sin(th)+lp*(dvy2+df2*vx2))/lp^2));
A_(3,:)=[ 0, 0, 0, 0, 0,-m0*vx2+mp*(vx2-vx2^2), 0, 0,a_317,0];
A_(4,:)=A_(3,:)*e;
A_(5,:)=A_(3,:)*hc2+...
[ 0, 0, 0, 0, 0, vx2*(h0*m0),0,2*dF2*lp*mp*sin(th)*(hp+lp-lp), ...
 mp*(dvy2*hp*sin(2*th)-g*hp*cos(2*th)-g*lp*cos(2*th)-dF2^2*lp^2*cos(2*th)-2*ddF2*lp^2*sin(th) ...
+dvy2*lp*sin(2*th)+dF2^2*lp^2-dth^2*lp^2-2*ddF2*hp*lp*sin(th)+dF2^2*hp*lp...
 -dth^2*hp*lp+co*dth*lp^2*sin(th)+df2*hp*vx2*sin(2*th)+df2*lp*vx2*sin(2*th)+co*dth*hp*lp*sin(th)),...
 -mp*(lp*(co+2*dth*sin(th))*(hp+lp-lp)+lp^2*sin(th)*(2*dth-co*sin(th)))];

%       1    2   3    4    5    6    7    8   9  10
%  X =  0,   0,  0,   0,   0, df2,   0,   0, th  0
% dX =  0;   0;  0;   0;dvy2;   0;dF2;ddF2;dth;  0
 Trans0=diag([vx1,1,1,1,vx2,1,1,1,1,1]);
 M_=Trans0*M_;
 A_=Trans0*A_;
 Acm=([M,zeros(8,2);zeros(2,10)]+M_)\([Acm0,zeros(8,2);zeros(2,10)]+A_);
 Bcm=([M,zeros(8,2);zeros(2,10)]+M_)\[Bcm0;zeros(2,1)];
 
 %% 增广状态量 并转变bi为vyi
 
 Trans=diag([1/vx1,1,1,1,1/vx2,1,1,1,1,1]);
 Ac=Trans*Acm;
 Bc=Trans*Bcm;
 
 %% 离散化线性模型
 [A,B]=c2d_zoh(Ac,Bc,Ts);             %离散化线性模型
 A0=A(1:8,1:8);
 A1=A(1:8,9:10);
 B0=B(1:8,1);
%       1   2    3    4   5    6    7    8   9  10
% dX=[dvy1;ddf1;dF1;ddF1;dvy2;ddf2;dF2;ddF2;th;dth];
%维度：10×1 
%% 进行状态估计
W=diag([20 10 20 1 20 20 20 1]);
Rho=diag([1.5 0.5])*0.0001;
Theta=(A1'*W*A1+Rho)\A1'*(state-A0*state0-B0*delta);

%% 保存状态量
th = RLS1(1,Theta(1),10,lambda);
dth0=(th-th0)/Ts;
th0=th;
% dth0 = RLS2(1,Theta(2),20,lambda);
% th0=Theta(1)*lambda+dth0*(1-lambda);dth0=Theta(2)*lambda+dth0*(1-lambda);
Theta(1)=th0;
Theta(2)=dth0;
state0=state;


end
function Fai = RLS1(fai_m1,Ym1,Nm,lambda)
persistent Pm_ Fai_ Ym fai_m
%初始赋值
if isempty(Pm_)
    Fai_=1e-10;
    Pm_=10*eye(Nm);
    Ym=ones(1,Nm)*1e-10;
    fai_m=ones(Nm,1);
end
%对fai_m 1xNm和 Ym 进行更新
fai_m(2:end)=fai_m(1:end-1);
Ym(2:end)=Ym(1:end-1);
fai_m(1)=fai_m1;
Ym(1)=Ym1;
%计算卡尔曼增益
K=Pm_*fai_m/(lambda+fai_m'*Pm_*fai_m);
%进行滤波
Fai=Fai_+(Ym-fai_m'*Fai_)*K;
%更新矩阵
Pm=1/lambda*(Pm_-K*fai_m'*Pm_);
Pm_=Pm;
Fai_=Fai;
end
function Fai = RLS2(fai_m1,Ym1,Nm,lambda)
persistent Pm_ Fai_ Ym fai_m
%初始赋值
if isempty(Pm_)
    Fai_=1e-10;
    Pm_=10*eye(Nm);
    Ym=ones(1,Nm)*1e-10;
    fai_m=ones(Nm,1);
end
%对fai_m 1xNm和 Ym 进行更新
fai_m(2:end)=fai_m(1:end-1);
Ym(2:end)=Ym(1:end-1);
fai_m(1)=fai_m1;
Ym(1)=Ym1;
%计算卡尔曼增益
K=Pm_*fai_m/(lambda+fai_m'*Pm_*fai_m);
%进行滤波
Fai=Fai_+(Ym-fai_m'*Fai_)*K;
%更新矩阵
Pm=1/lambda*(Pm_-K*fai_m'*Pm_);
Pm_=Pm;
Fai_=Fai;
end

%% 根据变量获取参数
function sim_param=getParam_SP(x)
%根据变量生成传输参数
TotMass=14462;
m1=x(1);%参数1
m0=TotMass-m1;
h0=x(2);%参数2
hp=x(3);%参数3
lp=x(4);%参数4
g=9.806;
coeff=x(5);%参数5
sim_param=[m0,m1,h0+0.77,hp+0.77,lp,g,coeff];
end

== matlab function ALGO_Tanker_new_5Pin_baseline/Theta_Estimation1 ==
  data: vx input; delta input; state input; Theta output
function Theta=Theta_Estimation(vx,delta,state)
%% 初始状态定义
%要记得设置本模块的采样时间哦
persistent Ts                            %采样时间
persistent th0 dth0 state0 lambda   %摆状态
if isempty(Ts)
   Ts=0.005;%采样时间
   %初始化状态量
   state0=zeros(2,1);
   lambda=0.995;
end
%% 定义动力学模型参数
persistent a b c d e                    %轴距纵向几何参数
persistent h1 h2 hc1 hc2                %质心至侧倾轴线距离
                                        %铰接点至侧倾轴线距离
persistent m1 m2 m1s m2s g;g=9.806;
persistent I1zz I1xx I1xz I2zz I2xx I2xz %惯性参量
persistent k1 k2 k3                      %线性轮胎模型参数
persistent kr1 kr2 c1 c2 k12             %悬架模型参数
persistent m0 mp h0 hp lp co             %摆模型参数
if isempty(a)
%SP模型，共5个参数拟合
% 参数 m1 h0 hp lp coeff
x=[10890,1.5,0.13,0.97,0.13];
sim_param=getParam_SP(x);
% sim_param=[m0,m1,h0+0.77,hp+0.77,lp,g,coeff];
m0=sim_param(1);
mp=sim_param(2);
h0=sim_param(3);
hp=sim_param(4);
lp=sim_param(5);
co=sim_param(7);
%车辆模型参数
L1=(5+6.27)/2;L2=(10.15+11.5)/2;       %轴距平均
a=1.385;b=L1-a;c=5.635-a;e=5.5;d=L2-e; %纵向几何
hm1s=1.02; %牵引车质心高度
hm2s=1.58; %50%充液率时半挂车质心高度
hhitch=1.1;%交接点高度
hroll1=0.2314;hroll2=0.9630;                     %侧倾中心高度
h1=hm1s-hroll1;h2=hm2s-hroll2;hc1=hhitch-hroll1;hc2=hhitch-hroll2;%高度几何
m1s=6310;m1=m1s+570+785*2;             %牵引车质量
% m2s=5925;m2=m2s+665*2;                 %半挂车空载质量
m2s=20387;m2=m2s+665*2;
I1xx=6879;I1xz=130;I1zz=19665;         %牵引车惯量
% I2xx=9960;I2xz=0;I2zz=179992;          %半挂车惯量
I2xx=34652;I2xz=0;I2zz=331380;
%轮胎模型参数
k1=-37e4;k2=-82e4;k3=-80e4;             %侧偏刚度
kr1=18.7e5;kr2=9.14e5;k12=68.3e5;             %侧倾刚度
c1=64.4e3;c2=197.7e3;                        %悬架等效阻尼
end
%% 定义线性动力学模型
vx1=vx(1);vx2=vx(2);dF2=state(8);
%线性车辆动力学模型
% M*dX = A0*X + B0*u
m14=-m1s*h1*c-I1xz;
m21=m1*vx1*hc1-m1s*h1*vx1;
m24=I1xx+2*m1s*h1^2-m1s*h1*hc1;
m55=m2*vx2*hc2-m2s*h2*vx2;
m58=I2xx+2*m2s*h2^2-m2s*h2*hc2;

M=[m1*vx1*c, I1zz, 0,   m14,     0,        0,   0,     0;
    m21,    -I1xz, 0,   m24,     0,        0,   0,     0;
   m1*vx1,      0, 0, -m1s*h1, m2*vx2,     0,   0, -m2s*h2;
     0,         0, 0,     0,  m2*vx2*e, -I2zz,  0, I2xz-m2s*h2*e;
     0,         0, 0,     0,    m55,    -I2xz,  0,    m58;
     1,    -c/vx1, 0, -hc1/vx1,  -1,   -e/vx2,  0, hc2/vx2;
     0,         0, 1,     0,     0,        0,   0,     0;
     0,         0, 0,     0,     0,        0,   1,     0   ];
 
 a11 = (c+a)*k1 + (c-b)*k2;
 a12 = a*(c+a)*k1/vx1 - b*(c-b)*k2/vx1 - m1*vx1*c;
 a22 = (a*k1-b*k2)*hc1/vx1 + (m1s*h1-m1*hc1)*vx1;
 a23 = m1s*g*h1 - kr1 -k12;
 a32 = (a*k1-b*k2)/vx1 - m1*vx1;
 a36 = -d*k3/vx2 - m2*vx2;
 a46 = -d*(e+d)*k3/vx2 - m2*vx2*e;
 a56 = (m2s*h2-m2*hc2)*vx2 - d*k3*hc2/vx2;
 a57 = m2s*g*h2 - kr2 -k12;
 %  X=   b1     df1    F1  dF1        b2  df2, F2   dF2 
 Acm0=[ a11,    a12,    0,   0,       0,   0,  0,    0;
   (k1+k2)*hc1, a22,  a23, -c1,       0,   0, k12,   0;
     k1+k2,     a32,    0,   0,      k3,  a36, 0,    0;
        0,       0,     0,   0, (e+d)*k3, a46, 0,    0;
        0,       0,    k12,  0,   k3*hc2, a56, a57, -c2;
        0,      -1,     0,   0,       0,   1,  0,    0;
        0,       0,     0,   1,       0,   0,  0,    0;
        0,       0,     0,   0,       0,   0,  0,    1   ];
    
 Bcm0=[-(c+a)*k1, -k1*hc1, -k1, 0, 0, 0, 0, 0]';

 %       1    2   3    4    5    6    7    8   9  10
%  X = vy1,  df1,F1, dF1, vy2, df2,  F2, dF2, th dth
% dX = dvy1;ddf1;dF1;ddF1;dvy2;ddf2;dF2;ddF2;dth;ddth ←M_
M_=zeros(10);
M_(9,9)=1;
M_(10,:)=[0,0,0,0,vx2/lp,0,0,hp/lp,0,1];
M_(3,:)=[0,0,0,0,(mp+m0)*vx2,0,(m0*h0+mp*(hp+lp))*dF2^2,-(m0+h0+mp*hp),0,mp*lp];
M_(4,:)=M_(3,:)*e;
M_(5,:)=M_(3,:)*hc2+...
[0,0,0,0,-(m0*h0+mp*hp)*vx2,0,0,(m0+h0^2+mp*hp^2),0,-mp*lp*hp];

A_=zeros(10);
A_(9,10)=1;
A_(10,:)=[0,0,0,0,0,-vx2/lp,0,0,-(hp/lp+1)*dF2^2-g/lp,-co];
A_(3,:)=[0,0,0,0,0,-(mp+m0)*vx2,0,0,0,0];
A_(4,:)=A_(3,:)*e;
A_(5,:)=A_(3,:)*hc2+...
[0,0,0,0,0,(m0*h0+mp*hp)*vx2,0,0,-mp*lp*g,0];
%       1    2   3    4    5    6    7    8   9  10
%  X =  0,   0,  0,   0,   0, df2,   0,   0, th  0
% dX =  0;   0;  0;   0;dvy2;   0;dF2;ddF2;dth;  0
 Acm=([M,zeros(8,2);zeros(2,10)]+M_)\([Acm0,zeros(8,2);zeros(2,10)]+A_);
 Bcm=([M,zeros(8,2);zeros(2,10)]+M_)\[Bcm0;zeros(2,1)];
 
 %% 增广状态量 并转变bi为vyi
 
 Trans=diag([1/vx1,1,1,1,1/vx2,1,1,1,1,1]);
 Ac=Trans*Acm;
 Bc=Trans*Bcm;
 %% 拆分状态矩阵，构造降阶状态观测器
 A11=Ac(1:8,1:8);
 A12=Ac(1:8,9:10);
 A21=Ac(9:10,1:8);
 A22=Ac(9:10,9:10);
 B1=Bc(1:8,1);
 B2=Bc(9:10,1);
 %% 离散化线性模型
  C=[1,1,0,0,1,5,0,0,0,0];
 coder.extrinsic('luenbergerObserver');
 L0=luenbergerObserver(Ac,C,-2*ones(1,10));
 L=zeros(10,1);
 L(1:10,1)=L0(1:10,1);
 [A,B]=c2d_zoh(Ac-L*C,[L,Bc],Ts);             %离散化线性模型

%       1   2    3    4   5    6    7    8   9  10
% dX=[dvy1;ddf1;dF1;ddF1;dvy2;ddf2;dF2;ddF2;th;dth];
%维度：10×1 
%% 进行状态估计
y=state;
state_est= A*state0 + B*[delta;state(7)];


%% 保存状态量
th=state_est(1);
% th = RLS1(1,Theta(1),50,lambda);
dth0=(th-th0)/Ts;
th0=th;
% dth0 = RLS2(1,Theta(2),20,lambda);
% th0=Theta(1)*lambda+dth0*(1-lambda);dth0=Theta(2)*lambda+dth0*(1-lambda);
Theta=zeros(2,1);
Theta(1)=th0;
Theta(2)=dth0;
state0=state_est;


end

%% 根据变量获取参数
function sim_param=getParam_SP(x)
%根据变量生成传输参数
TotMass=14462;
m1=x(1);%参数1
m0=TotMass-m1;
h0=x(2);%参数2
hp=x(3);%参数3
lp=x(4);%参数4
g=9.806;
coeff=x(5);%参数5
sim_param=[m0,m1,h0+0.77,hp+0.77,lp,g,coeff];
end
% function Fai = RLS1(fai_m1,Ym1,Nm,lambda)
% persistent Pm_ Fai_ Ym fai_m
% %初始赋值
% if isempty(Pm_)
%     Fai_=1e-10;
%     Pm_=10*eye(Nm);
%     Ym=ones(1,Nm)*1e-10;
%     fai_m=ones(Nm,1);
% end
% %对fai_m 1xNm和 Ym 进行更新
% fai_m(2:end)=fai_m(1:end-1);
% Ym(2:end)=Ym(1:end-1);
% fai_m(1)=fai_m1;
% Ym(1)=Ym1;
% %计算卡尔曼增益
% K=Pm_*fai_m/(lambda+fai_m'*Pm_*fai_m);
% %进行滤波
% Fai=Fai_+(Ym-fai_m'*Fai_)*K;
% %更新矩阵
% Pm=1/lambda*(Pm_-K*fai_m'*Pm_);
% Pm_=Pm;
% Fai_=Fai;
% end
% function Fai = RLS2(fai_m1,Ym1,Nm,lambda)
% persistent Pm_ Fai_ Ym fai_m
% %初始赋值
% if isempty(Pm_)
%     Fai_=1e-10;
%     Pm_=10*eye(Nm);
%     Ym=ones(1,Nm)*1e-10;
%     fai_m=ones(Nm,1);
% end
% %对fai_m 1xNm和 Ym 进行更新
% fai_m(2:end)=fai_m(1:end-1);
% Ym(2:end)=Ym(1:end-1);
% fai_m(1)=fai_m1;
% Ym(1)=Ym1;
% %计算卡尔曼增益
% K=Pm_*fai_m/(lambda+fai_m'*Pm_*fai_m);
% %进行滤波
% Fai=Fai_+(Ym-fai_m'*Fai_)*K;
% %更新矩阵
% Pm=1/lambda*(Pm_-K*fai_m'*Pm_);
% Pm_=Pm;
% Fai_=Fai;
% end

== matlab function ALGO_Tanker_new_5Pin_baseline/MyEstimationMethod ==
  data: vx input; delta input; ddF2 input; dvy2 input; state input; Theta output
function Theta=Theta_Estimation(vx,delta,ddF2,dvy2,state)
%% 初始状态定义
%要记得设置本模块的采样时间哦
persistent Ts                             %采样时间
persistent th0 dth0 state0 lambda   %摆状态
if isempty(th0)
    Ts=0.005;
   th0=0;dth0=0; 
   state0=zeros(8,1);
   lambda=0.995;
end
%% 定义动力学模型参数
persistent a b c d e                    %轴距纵向几何参数
persistent h1 h2 hc1 hc2                %质心至侧倾轴线距离
                                        %铰接点至侧倾轴线距离
persistent m1 m2 m1s m2s g;g=9.806;
persistent I1zz I1xx I1xz I2zz I2xx I2xz %惯性参量
persistent k1 k2 k3                      %线性轮胎模型参数
persistent kr1 kr2 c1 c2 k12             %悬架模型参数
persistent m0 mp h0 hp lp co             %摆模型参数
if isempty(a)
%SP模型，共5个参数拟合
% 参数 m1 h0 hp lp coeff
x=[10890,1.5,0.13,0.97,0.13];
sim_param=getParam_SP(x);
% sim_param=[m0,m1,h0+0.77,hp+0.77,lp,g,coeff];
m0=sim_param(1);
mp=sim_param(2);
h0=sim_param(3);
hp=sim_param(4);
lp=sim_param(5);
co=sim_param(7);
%车辆模型参数
L1=(5+6.27)/2;L2=(10.15+11.5)/2;       %轴距平均
a=1.385;b=L1-a;c=5.635-a;e=5.5;d=L2-e; %纵向几何
hm1s=1.02; %牵引车质心高度
hm2s=1.58; %50%充液率时半挂车质心高度
hhitch=1.1;%交接点高度
hroll1=0.2314;hroll2=0.9630;                     %侧倾中心高度
h1=hm1s-hroll1;h2=hm2s-hroll2;hc1=hhitch-hroll1;hc2=hhitch-hroll2;%高度几何
m1s=6310;m1=m1s+570+785*2;             %牵引车质量
% m2s=5925;m2=m2s+665*2;                 %半挂车空载质量
m2s=20387;m2=m2s+665*2;
I1xx=6879;I1xz=130;I1zz=19665;         %牵引车惯量
% I2xx=9960;I2xz=0;I2zz=179992;          %半挂车惯量
I2xx=34652;I2xz=0;I2zz=331380;
%轮胎模型参数
k1=-37e4;k2=-82e4;k3=-80e4;             %侧偏刚度
kr1=18.7e5;kr2=9.14e5;k12=68.3e5;             %侧倾刚度
c1=64.4e3;c2=197.7e3;                        %悬架等效阻尼
end
%% 定义线性动力学模型
df2=state0(6);
dF2=state0(8);
vx1=vx(1);vx2=vx(2);
%线性车辆动力学模型
% M*dX = A0*X + B0*u
m14=-m1s*h1*c-I1xz;
m21=m1*vx1*hc1-m1s*h1*vx1;
m24=I1xx+2*m1s*h1^2-m1s*h1*hc1;
m55=m2*vx2*hc2-m2s*h2*vx2;
m58=I2xx+2*m2s*h2^2-m2s*h2*hc2;
m410=-mp*lp*e;

M=[m1*vx1*c, I1zz, 0,   m14,     0,        0,   0,     0,     0,    0;
    m21,    -I1xz, 0,   m24,     0,        0,   0,     0,     0,    0;
   m1*vx1,      0, 0, -m1s*h1, m2*vx2,     0,   0, -m2s*h2,   0, -mp*lp;
     0,         0, 0,     0,  m2*vx2*e, -I2zz,  0, I2xz-m2s*h2*e,0,m410;
     0,         0, 0,     0,    m55,    -I2xz,  0,    m58,    0,    0;
     1,    -c/vx1, 0, -hc1/vx1,  -1,   -e/vx2,  0, hc2/vx2,   0,    0;
     0,         0, 1,     0,     0,        0,   0,     0,     0,    0;
     0,         0, 0,     0,     0,        0,   1,     0,     0,    0;
     0,         0, 0,     0, -vx2/lp,      0,   0, h2/lp,    co,    1;
     0,         0, 0,     0,     0,        0,   0,     0,     1,    0];
 
 a11 = (c+a)*k1 + (c-b)*k2;
 a12 = a*(c+a)*k1/vx1 - b*(c-b)*k2/vx1 - m1*vx1*c;
 a22 = (a*k1-b*k2)*hc1/vx1 + (m1s*h1-m1*hc1)*vx1;
 a23 = m1s*g*h1 - kr1 -k12;
 a32 = (a*k1-b*k2)/vx1 - m1*vx1;
 a36 = -d*k3/vx2 - m2*vx2;
 a46 = -d*(e+d)*k3/vx2 - m2*vx2*e;
 a56 = (m2s*h2-m2*hc2)*vx2 - d*k3*hc2/vx2;
 a57 = m2s*g*h2 - kr2 -k12;
 %  X=   b1     df1    F1  dF1        b2  df2, F2   dF2 
 Acm0=[ a11,    a12,    0,   0,       0,   0,  0,    0,   0,   0;
   (k1+k2)*hc1, a22,  a23, -c1,       0,   0, k12,   0,   0,   0;
     k1+k2,     a32,    0,   0,      k3,  a36, 0,    0,   0,   0;
        0,       0,     0,   0, (e+d)*k3, a46, 0,    0,   0,   0;
        0,       0,    k12,  0,  e*k3*h2, a56, a57, -c2, mp*lp*g,0;
        0,      -1,     0,   0,       0,   1,  0,    0,   0,   0;
        0,       0,     0,   1,       0,   0,  0,    0,   0,   0;
        0,       0,     0,   0,       0,   0,  0,    1,   0,   0;
        0,       0,     0,   0,       0,vx2/lp,0,    0, g/lp,  0;
        0,       0,     0,   0,       0,   0,  0,    0,   0,   1];
    
 Bcm0=[-(c+a)*k1, -k1*hc1, -k1, 0, 0, 0, 0, 0, 0, 0]';


 Acm=M\Acm0;
 Bcm=M\Bcm0;
 
 %% 增广状态量 并转变bi为vyi
 
 Trans=diag([1/vx1,1,1,1,1/vx2,1,1,1,1,1]);
 Ac=Trans*Acm;
 Bc=Trans*Bcm;
 
 %% 离散化线性模型
 [A,B]=c2d_zoh(Ac,Bc,Ts);             %离散化线性模型
 A0=A(1:8,1:8);
 A1=A(1:8,9:10);
 B0=B(1:8,1);
%       1   2    3    4   5    6    7    8   9  10
% dX=[dvy1;ddf1;dF1;ddF1;dvy2;ddf2;dF2;ddF2;th;dth];
%维度：10×1 
%% 进行状态估计
W=diag([10 10 1 1 10 10 10 1]);
Rho=diag([0.5 0.5])*0.003;
Theta=(A1'*W*A1+Rho)\A1'*(state-A0*state0-B0*delta);

%% 保存状态量
th = RLS1(1,Theta(1),20,lambda);
dth0=(th-th0)/Ts;
th0=th;
% dth0 = RLS2(1,Theta(2),20,lambda);
% th0=Theta(1)*lambda+dth0*(1-lambda);dth0=Theta(2)*lambda+dth0*(1-lambda);
Theta(1)=-th0;
Theta(2)=-dth0;
state0=state;


end
function Fai = RLS1(fai_m1,Ym1,Nm,lambda)
persistent Pm_ Fai_ Ym fai_m
%初始赋值
if isempty(Pm_)
    Fai_=1e-10;
    Pm_=10*eye(Nm);
    Ym=ones(1,Nm)*1e-10;
    fai_m=ones(Nm,1);
end
%对fai_m 1xNm和 Ym 进行更新
fai_m(2:end)=fai_m(1:end-1);
Ym(2:end)=Ym(1:end-1);
fai_m(1)=fai_m1;
Ym(1)=Ym1;
%计算卡尔曼增益
K=Pm_*fai_m/(lambda+fai_m'*Pm_*fai_m);
%进行滤波
Fai=Fai_+(Ym-fai_m'*Fai_)*K;
%更新矩阵
Pm=1/lambda*(Pm_-K*fai_m'*Pm_);
Pm_=Pm;
Fai_=Fai;
end
function Fai = RLS2(fai_m1,Ym1,Nm,lambda)
persistent Pm_ Fai_ Ym fai_m
%初始赋值
if isempty(Pm_)
    Fai_=1e-10;
    Pm_=10*eye(Nm);
    Ym=ones(1,Nm)*1e-10;
    fai_m=ones(Nm,1);
end
%对fai_m 1xNm和 Ym 进行更新
fai_m(2:end)=fai_m(1:end-1);
Ym(2:end)=Ym(1:end-1);
fai_m(1)=fai_m1;
Ym(1)=Ym1;
%计算卡尔曼增益
K=Pm_*fai_m/(lambda+fai_m'*Pm_*fai_m);
%进行滤波
Fai=Fai_+(Ym-fai_m'*Fai_)*K;
%更新矩阵
Pm=1/lambda*(Pm_-K*fai_m'*Pm_);
Pm_=Pm;
Fai_=Fai;
end

%% 根据变量获取参数
function sim_param=getParam_SP(x)
%根据变量生成传输参数
TotMass=14462;
m1=x(1);%参数1
m0=TotMass-m1;
h0=x(2);%参数2
hp=x(3);%参数3
lp=x(4);%参数4
g=9.806;
coeff=x(5);%参数5
sim_param=[m0,m1,h0+0.77,hp+0.77,lp,g,coeff];
end

== matlab function ALGO_Tanker_new_5Pin_baseline/LuenbergerSISOestimation ==
  data: vx input; delta input; state input; Theta output
function Theta=Theta_Estimation(vx,delta,state)
%% 初始状态定义
%要记得设置本模块的采样时间哦
persistent Ts                            %采样时间
persistent th0 dth0 state0 lambda   %摆状态
if isempty(Ts)
   Ts=0.005;%采样时间
   %初始化状态量
   th0=0;dth0=0; 
   state0=zeros(10,1);
   lambda=0.995;
end
%% 定义动力学模型参数
persistent a b c d e                    %轴距纵向几何参数
persistent h1 h2 hc1 hc2                %质心至侧倾轴线距离
                                        %铰接点至侧倾轴线距离
persistent m1 m2 m1s m2s g;g=9.806;
persistent I1zz I1xx I1xz I2zz I2xx I2xz %惯性参量
persistent k1 k2 k3                      %线性轮胎模型参数
persistent kr1 kr2 c1 c2 k12             %悬架模型参数
persistent m0 mp h0 hp lp co             %摆模型参数
if isempty(a)
%SP模型，共5个参数拟合
% 参数 m1 h0 hp lp coeff
x=[10890,1.5,0.13,0.97,0.13];
sim_param=getParam_SP(x);
% sim_param=[m0,m1,h0+0.77,hp+0.77,lp,g,coeff];
m0=sim_param(1);
mp=sim_param(2);
h0=sim_param(3);
hp=sim_param(4);
lp=sim_param(5);
co=sim_param(7);
%车辆模型参数
L1=(5+6.27)/2;L2=(10.15+11.5)/2;       %轴距平均
a=1.385;b=L1-a;c=5.635-a;e=5.5;d=L2-e; %纵向几何
hm1s=1.02; %牵引车质心高度
hm2s=1.58; %50%充液率时半挂车质心高度
hhitch=1.1;%交接点高度
hroll1=0.2314;hroll2=0.9630;                     %侧倾中心高度
h1=hm1s-hroll1;h2=hm2s-hroll2;hc1=hhitch-hroll1;hc2=hhitch-hroll2;%高度几何
m1s=6310;m1=m1s+570+785*2;             %牵引车质量
% m2s=5925;m2=m2s+665*2;                 %半挂车空载质量
m2s=20387;m2=m2s+665*2;
I1xx=6879;I1xz=130;I1zz=19665;         %牵引车惯量
% I2xx=9960;I2xz=0;I2zz=179992;          %半挂车惯量
I2xx=9960;I2xz=0;I2zz=331380;
%轮胎模型参数
k1=-37e4;k2=-82e4;k3=-80e4;             %侧偏刚度
kr1=18.7e5;kr2=9.14e5;k12=68.3e5;             %侧倾刚度
c1=64.4e3;c2=197.7e3;                        %悬架等效阻尼
end
%% 定义线性动力学模型
vx1=vx(1);vx2=vx(2);dF2=state(8);
%线性车辆动力学模型
% M*dX = A0*X + B0*u
m14=-m1s*h1*c-I1xz;
m21=m1*vx1*hc1-m1s*h1*vx1;
m24=I1xx+2*m1s*h1^2-m1s*h1*hc1;
m55=m2*vx2*hc2-m2s*h2*vx2;
m58=I2xx+2*m2s*h2^2-m2s*h2*hc2;

M=[m1*vx1*c, I1zz, 0,   m14,     0,        0,   0,     0;
    m21,    -I1xz, 0,   m24,     0,        0,   0,     0;
   m1*vx1,      0, 0, -m1s*h1, m2*vx2,     0,   0, -m2s*h2;
     0,         0, 0,     0,  m2*vx2*e, -I2zz,  0, I2xz-m2s*h2*e;
     0,         0, 0,     0,    m55,    -I2xz,  0,    m58;
     1,    -c/vx1, 0, -hc1/vx1,  -1,   -e/vx2,  0, hc2/vx2;
     0,         0, 1,     0,     0,        0,   0,     0;
     0,         0, 0,     0,     0,        0,   1,     0   ];
 
 a11 = (c+a)*k1 + (c-b)*k2;
 a12 = a*(c+a)*k1/vx1 - b*(c-b)*k2/vx1 - m1*vx1*c;
 a22 = (a*k1-b*k2)*hc1/vx1 + (m1s*h1-m1*hc1)*vx1;
 a23 = m1s*g*h1 - kr1 -k12;
 a32 = (a*k1-b*k2)/vx1 - m1*vx1;
 a36 = -d*k3/vx2 - m2*vx2;
 a46 = -d*(e+d)*k3/vx2 - m2*vx2*e;
 a56 = (m2s*h2-m2*hc2)*vx2 - d*k3*hc2/vx2;
 a57 = m2s*g*h2 - kr2 -k12;
 %  X=   b1     df1    F1  dF1        b2  df2, F2   dF2 
 Acm0=[ a11,    a12,    0,   0,       0,   0,  0,    0;
   (k1+k2)*hc1, a22,  a23, -c1,       0,   0, k12,   0;
     k1+k2,     a32,    0,   0,      k3,  a36, 0,    0;
        0,       0,     0,   0, (e+d)*k3, a46, 0,    0;
        0,       0,    k12,  0,   k3*hc2, a56, a57, -c2;
        0,      -1,     0,   0,       0,   1,  0,    0;
        0,       0,     0,   1,       0,   0,  0,    0;
        0,       0,     0,   0,       0,   0,  0,    1   ];
    
 Bcm0=[-(c+a)*k1, -k1*hc1, -k1, 0, 0, 0, 0, 0]';

 %       1    2   3    4    5    6    7    8   9  10
%  X = vy1,  df1,F1, dF1, vy2, df2,  F2, dF2, th dth
% dX = dvy1;ddf1;dF1;ddF1;dvy2;ddf2;dF2;ddF2;dth;ddth ←M_
M_=zeros(10);
M_(9,9)=1;
M_(10,:)=[0,0,0,0,vx2/lp,0,0,hp/lp,0,1];
M_(3,:)=[0,0,0,0,(mp+m0)*vx2,0,(m0*h0+mp*(hp+lp))*dF2^2,-(m0+h0+mp*hp),0,mp*lp];
M_(4,:)=M_(3,:)*e;
M_(5,:)=M_(3,:)*hc2+...
[0,0,0,0,-(m0*h0+mp*hp)*vx2,0,0,(m0+h0^2+mp*hp^2),0,-mp*lp*hp];

A_=zeros(10);
A_(9,10)=1;
A_(10,:)=[0,0,0,0,0,-vx2/lp,0,0,-(hp/lp+1)*dF2^2-g/lp,-co];
A_(3,:)=[0,0,0,0,0,-(mp+m0)*vx2,0,0,0,0];
A_(4,:)=A_(3,:)*e;
A_(5,:)=A_(3,:)*hc2+...
[0,0,0,0,0,(m0*h0+mp*hp)*vx2,0,0,-mp*lp*g,0];
%       1    2   3    4    5    6    7    8   9  10
%  X =  0,   0,  0,   0,   0, df2,   0,   0, th  0
% dX =  0;   0;  0;   0;dvy2;   0;dF2;ddF2;dth;  0
 Acm=([M,zeros(8,2);zeros(2,10)]+M_)\([Acm0,zeros(8,2);zeros(2,10)]+A_);
 Bcm=([M,zeros(8,2);zeros(2,10)]+M_)\[Bcm0;zeros(2,1)];
 
 %% 增广状态量 并转变bi为vyi
 
 Trans=diag([1/vx1,1,1,1,1/vx2,1,1,1,1,1]);
 Ac=Trans*Acm;
 Bc=Trans*Bcm;
 
 %% 离散化线性模型
  C=[1,1,3,3,1,1,20,20,0,0];
 coder.extrinsic('luenbergerObserver');
 L0=luenbergerObserver(Ac,C,-5*ones(1,10));
 L=zeros(10,1);
 L(1:10,1)=L0(1:10,1);
 [A,B]=c2d_zoh(Ac-L*C,[L,Bc],Ts);             %离散化线性模型

%       1   2    3    4   5    6    7    8   9  10
% dX=[dvy1;ddf1;dF1;ddF1;dvy2;ddf2;dF2;ddF2;th;dth];
%维度：10×1 
%% 进行状态估计
state_est= A*state0 + B*[delta;state(7)];


%% 保存状态量
th=state_est(9);
% th = RLS1(1,Theta(1),50,lambda);
dth0=(th-th0)/Ts;
th0=th;
% dth0 = RLS2(1,Theta(2),20,lambda);
% th0=Theta(1)*lambda+dth0*(1-lambda);dth0=Theta(2)*lambda+dth0*(1-lambda);
Theta=zeros(2,1);
Theta(1)=th0;
Theta(2)=dth0;
state0=state_est;


end

%% 根据变量获取参数
function sim_param=getParam_SP(x)
%根据变量生成传输参数
TotMass=14462;
m1=x(1);%参数1
m0=TotMass-m1;
h0=x(2);%参数2
hp=x(3);%参数3
lp=x(4);%参数4
g=9.806;
coeff=x(5);%参数5
sim_param=[m0,m1,h0+0.77,hp+0.77,lp,g,coeff];
end
% function Fai = RLS1(fai_m1,Ym1,Nm,lambda)
% persistent Pm_ Fai_ Ym fai_m
% %初始赋值
% if isempty(Pm_)
%     Fai_=1e-10;
%     Pm_=10*eye(Nm);
%     Ym=ones(1,Nm)*1e-10;
%     fai_m=ones(Nm,1);
% end
% %对fai_m 1xNm和 Ym 进行更新
% fai_m(2:end)=fai_m(1:end-1);
% Ym(2:end)=Ym(1:end-1);
% fai_m(1)=fai_m1;
% Ym(1)=Ym1;
% %计算卡尔曼增益
% K=Pm_*fai_m/(lambda+fai_m'*Pm_*fai_m);
% %进行滤波
% Fai=Fai_+(Ym-fai_m'*Fai_)*K;
% %更新矩阵
% Pm=1/lambda*(Pm_-K*fai_m'*Pm_);
% Pm_=Pm;
% Fai_=Fai;
% end
% function Fai = RLS2(fai_m1,Ym1,Nm,lambda)
% persistent Pm_ Fai_ Ym fai_m
% %初始赋值
% if isempty(Pm_)
%     Fai_=1e-10;
%     Pm_=10*eye(Nm);
%     Ym=ones(1,Nm)*1e-10;
%     fai_m=ones(Nm,1);
% end
% %对fai_m 1xNm和 Ym 进行更新
% fai_m(2:end)=fai_m(1:end-1);
% Ym(2:end)=Ym(1:end-1);
% fai_m(1)=fai_m1;
% Ym(1)=Ym1;
% %计算卡尔曼增益
% K=Pm_*fai_m/(lambda+fai_m'*Pm_*fai_m);
% %进行滤波
% Fai=Fai_+(Ym-fai_m'*Fai_)*K;
% %更新矩阵
% Pm=1/lambda*(Pm_-K*fai_m'*Pm_);
% Pm_=Pm;
% Fai_=Fai;
% end
